simulink model "schSegwayArduino_2018a"  (R2018b)
settings: Solver=FixedStepDiscrete  StartTime=0.0  StopTime=inf  FixedStep=TECH  RelTol=1e-3  EnableMultiTasking=on
PreLoadFcn:
  | file:///C:/Users/maitrise/Documents/Elie/segwayEtudiant/segwayEtudiant/CzLeftRight.mat
InitFcn:
  | load CLeftRight.mat;
  | load  Kplace.mat
values from neighbouring files (symbols this model uses):
  K = [-22.0083946552 -0.385164851676 -3.66015572739 -0.971821179518]    [Kplace.mat]    (also in convertToParallelCells.m = 0; paralellCells.m = 0; programme_segway_etudiant.m = place(A,BUm,poles_BF))
  TECH = min(t(2:end)-t(1:(end-1)))    [drawScopeData.m]    (also in programme_segway_etudiant.m = 0.005)
  tfCLeftRight = tf(NumC,DenC)    [programme_segway_etudiant.m]
undefined symbols (not defined in the file or in its folder): denZ, numZ
libraries: arduinolib x7, cstblocks x1
settings Model: SimulationMode=external  ExtModeTrigDuration=2  Creator=KSURCT General  LastModifiedBy=maitrise
settings OptimizationCC: DefaultUnderspecifiedDataType=single  EnhancedBackFolding=on  PassReuseOutputArgsThreshold=0  MaxStackSize=64  OptimizeBlockOrder=speed  DifferentSizesBufferReuse=on  OptimizationCustomize=off
settings DebuggingCC: ParameterTunabilityLossMsg=error
settings HardwareCC: ProdBitPerPointer=32  ProdBitPerSizeT=32  ProdBitPerPtrDiffT=32  ProdLargestAtomicInteger=Long  ProdLargestAtomicFloat=Double  ProdWordSize=32  ProdHWDeviceType=ARM Compatible->ARM Cortex  UseEmbeddedCoderFeatures=off  UseSimulinkCoderFeatures=off
settings SFSimCC: MATLABDynamicMemAlloc=off
settings RTWCC: SystemTargetFile=ert.tlc  HardwareBoard=Arduino Due  TemplateMakefile=ert_default_tmf  GenerateReport=on  Toolchain=Arduino ARM  BuildConfiguration=Faster Runs  LaunchReport=on
settings CodeAppCC: ForceParamTrailComments=on  OperatorAnnotations=on  MangleLength=10
settings ERTTargetCC: ERTCustomFileBanners=off  SupportContinuousTime=on  SupportNonInlinedSFcns=on  RemoveResetFunc=off  SupportVariableSizeSignals=on  ModelStepFunctionPrototypeControlCompliant=off

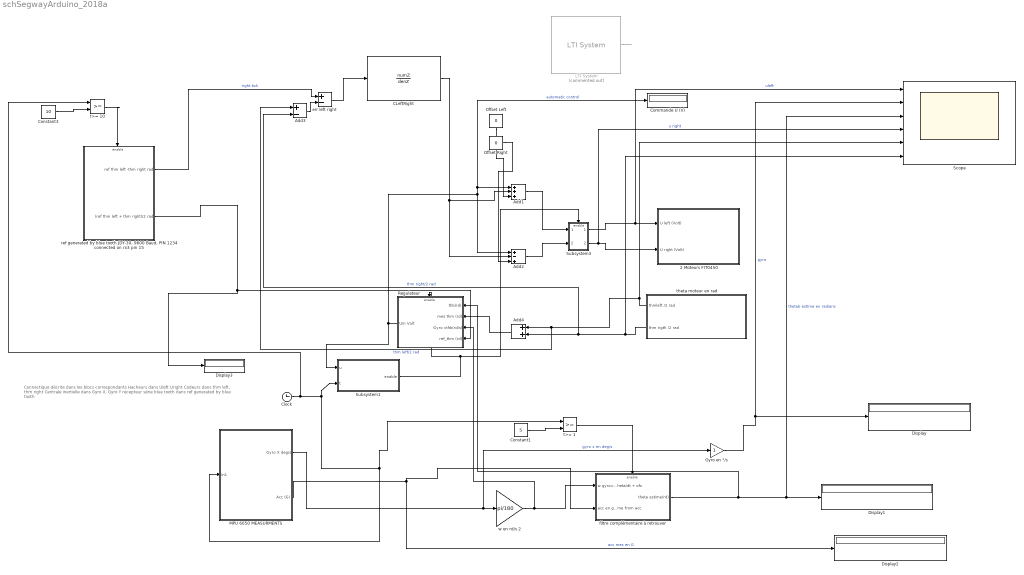
== system schSegwayArduino_2018a ==
  note: Connectique décrite dans les blocs correspondants
      | Hacheurs dans Uleft Uright
      | Codeurs dans thm left, thm right
      | Centrale inertielle dans Gyro X, Gyro Y
      | récepteur série blue tooth dans ref generated by blue tooth
  2 Moteurs FIT0450 : Subsystem
  Add1 : Sum  Inputs=+++
  Add2 : Sum  Inputs=+-+
  Add3 : Sum  Inputs=+-
  Add4 : Sum
  CLeftRight : DiscreteTransferFcn  Numerator=numZ  Denominator=denZ  SampleTime=TECH  mask(Tustin){tfP=tfCLeftRight, Tech=TECH}
      mask prompts: tfP "transfer Function F(p)"; Tech "Sample Time(s)"
      mask help:
      | discrete approximation (Tustin) of continuous transfer function
      | p -> 2/Te (z-1)/(z+1)
      mask init:
      | tfZ=c2d(tfP,Tech,'tustin');
      | [numZ,denZ]=tfdata(tfZ,'vector');
      mask Display: disp('F(p) \nTustin approx')
  Clock : Clock
  Commande U (V) : Display
  Constant1 : Constant  Value=5
  Constant3 : Constant  Value=10
  Display{,1..3} (4 alike) : Display
  Gyro en °/s : Gain
  LTI System : cstblocks/LTI System  Commented=on  sys=tf([1.42e2,2.36e3],[1,78])  IC=[]
  MPU 6050 MEASURMENTS : Subsystem
  "Offset Left " : Constant  Value=0
  Offset Right : Constant  Value=0
  Regulateur : Subsystem  TreatAsAtomicUnit=on
      settings: AttributesFormatString=REGULATEUR
  Scope : Scope  NumInputPorts=6
  Subsystem1 : Subsystem
  Subsystem3 : Subsystem
  err left right : Sum  Inputs=+-
  filtre complémentaire à retrouver : Subsystem
  "ref generated by blue tooth JDY-30, 9600 Baud, PIN 1234 connected on rx3 pin 15" : Subsystem
  t>= 1 : RelationalOperator  OutDataTypeStr=boolean  RndMeth=Simplest
  t>= 10 : RelationalOperator  OutDataTypeStr=boolean  RndMeth=Simplest
  theta moteur en rad : Subsystem
  w en rd/s 2 : Gain  Gain=pi/180
  wires:
  Subsystem1/1(enable) -> Subsystem3/Enable, Regulateur/Enable
  Add1/1 -> Subsystem3/1(In1)
  Add2/1 -> Subsystem3/2(In2)
  Subsystem3/1(Commande (V)) -> Scope/1, 2 Moteurs FIT0450/1(U left (Volt))  "uleft"
  Subsystem3/2(Commande (V)1) -> Scope/4, 2 Moteurs FIT0450/2(U right (Volt))  "u right"
  "ref generated by blue tooth JDY-30, 9600 Baud, PIN 1234 connected on rx3 pin 15"/2((ref thm left + thm right)/2 rad) -> Display3/1, Regulateur/4("ref_thm (rd) ")
  "ref generated by blue tooth JDY-30, 9600 Baud, PIN 1234 connected on rx3 pin 15"/1(ref thm left -thm right rad) -> err left right/1  "right tick"
  Regulateur/1(Um Volt) -> Commande U (V)/1, Add1/1, Add2/1, Subsystem1/1(u)  "automatic control"
  Clock/1 -> t>= 10/1, Subsystem1/2(t), t>= 1/1, MPU 6050 MEASURMENTS/1(In1)
  Gyro en °/s/1 -> Scope/2, Display/1  "gyro"
  CLeftRight/1 -> Add1/2, Add2/2
  t>= 10/1 -> "ref generated by blue tooth JDY-30, 9600 Baud, PIN 1234 connected on rx3 pin 15"/Enable
  Constant3/1 -> t>= 10/2
  theta moteur en rad/1(thmleft /2 rad) -> Scope/5, Add3/1, Add4/1  "thm left/2 rad"
  theta moteur en rad/2(thm rigth /2 rad) -> Scope/6, Add3/2, Add4/2  "thm right/2 rad"
  Add4/1 -> Regulateur/2(mes thm (rd))
  Add3/1 -> err left right/2
  "Offset Left "/1 -> Add1/3
  Offset Right/1 -> Add2/3
  filtre complémentaire à retrouver/1(theta estime(rd)) -> Regulateur/1(thb(rd)), Scope/3, Display1/1  "thetab estime en radians"
  MPU 6050 MEASURMENTS/1("Gyro X deg/s  ") -> Gyro en °/s/1, w en rd/s 2/1  "gyro x en deg/s"
  MPU 6050 MEASURMENTS/2(Acc (G)) -> Display2/1, filtre complémentaire à retrouver/2("acc en g = theta estime from acc ")  "acc mes en G"
  w en rd/s 2/1 -> Regulateur/3(Gyro vthb(rd/s)), filtre complémentaire à retrouver/1(w gyro=dtheta/dt + ofs)
  Constant1/1 -> t>= 1/2
  t>= 1/1 -> filtre complémentaire à retrouver/Enable
  LTI System/1 -> ?
  err left right/1 -> CLeftRight/1
  ? -> LTI System/1

== system schSegwayArduino_2018a/2 Moteurs FIT0450 ==
  note: CONNECTIQUE
      | Batterie de puissance : power Banc VoltCraft
      | brancher 2 resistances de 150 ohms 1/4 de watt en parallele sur la sortie 5V pour empecher la mise en pause
      | Hacheurs : MC33926 2,5 A et marche a 5V
      | Moteur droit FIT 0450U : Km=0,277 Nm/A , R=2,8ohm, Im=6e-3 kg m2 , fm =0.01 Nm/(rd/s)
      | Borne 39 Due sur In1 du pont en H
      | Borne 38 Due sur In2 du pont en H
      | Moteur gauche FIT 0450U
      | Borne 35 Due sur In1 du pont en H
      | Borne 34 Due sur In2 du pont en H
      | Moteurs droit et gauche
      | Fil noir moteurs sur out2 des ponts en H
      | Fil rouge moteurs sur out 1 des ponts en H
      | Gnd Due sur borne - (logique )
      | Gnd Alim Puissance sur borne - (puissance)
      | Vcc Alim Puissance 5V sur borne +, pas le 5v de la due, le 5v de puissance !
      | Codeur incremental moteur gauche (120.32 pas par tour)
      | fil rouge codeur sur 3,3V due ( surtout pas sur 5V : ATTENTION !... .)
      | fil noir codeur sur gnd due
      | fil bleu codeur sur borne 7 due
      | fil vert codeur sur borne 6 due
      | Codeur incremental moteur droit (120.32 pas par tour)
      | fil rouge codeur sur 3,3V due ( surtout pas sur 5V : ATTENTION !... .)
      | fil noir codeur sur gnd due
      | fil bleu codeur sur borne 4 due
      | fil vert codeur sur borne 3 due
  U left (Volt) : Inport
  U right (Volt) : Inport  Port=2
  Apply Command Pwm : Subsystem
  wires:
  U left (Volt)/1 -> Apply Command Pwm/1(U left (Volt))
  U right (Volt)/1 -> Apply Command Pwm/2(U right (Volt))

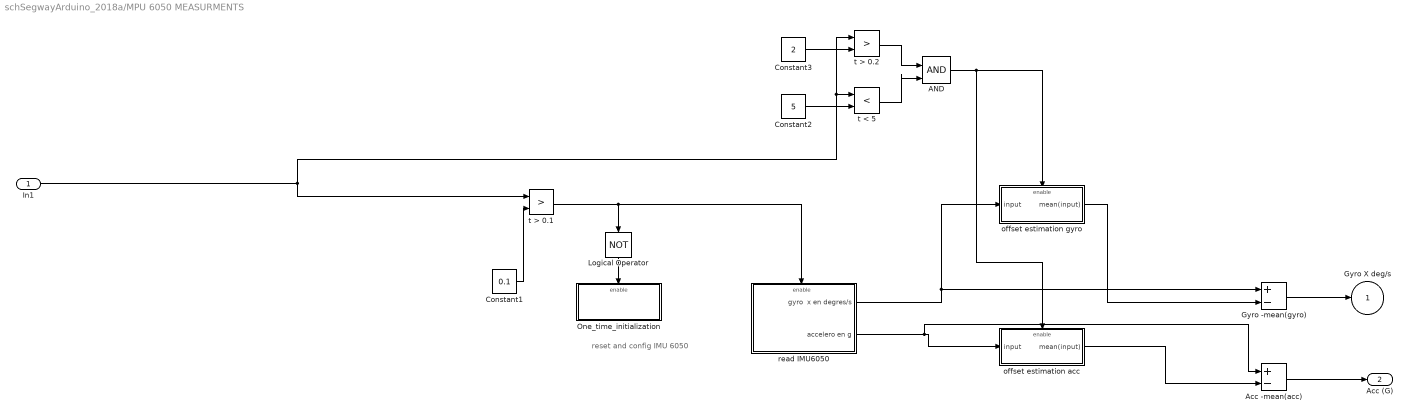
== system schSegwayArduino_2018a/MPU 6050 MEASURMENTS ==
  note: reset and config
      | IMU 6050
  In1 : Inport
  AND : Logic  IconShape=distinctive  AllPortsSameDT=off  OutDataTypeStr=boolean
  Acc -mean(acc) : Sum  Inputs=+-
  Constant1 : Constant  Value=0.1
  Constant2 : Constant  Value=5
  Constant3 : Constant  Value=2
  Gyro -mean(gyro) : Sum  Inputs=+-
  Logical Operator : Logic  Operator=NOT  AllPortsSameDT=off  OutDataTypeStr=boolean
  One_time_initialization : Subsystem  TreatAsAtomicUnit=on
  offset estimation acc : Subsystem  TreatAsAtomicUnit=on
  offset estimation gyro : Subsystem  TreatAsAtomicUnit=on
  read IMU6050 : Subsystem  TreatAsAtomicUnit=on
  t < 5 : RelationalOperator  Operator=<  OutDataTypeStr=boolean  RndMeth=Simplest
  t > 0.1 : RelationalOperator  Operator=>  OutDataTypeStr=boolean  RndMeth=Simplest
  t > 0.2 : RelationalOperator  Operator=>  OutDataTypeStr=boolean  RndMeth=Simplest
  "Gyro X deg/s  " : Outport
  Acc (G) : Outport  Port=2
  wires:
  t < 5/1 -> AND/2
  Logical Operator/1 -> One_time_initialization/Enable
  t > 0.1/1 -> read IMU6050/Enable, Logical Operator/1
  Gyro -mean(gyro)/1 -> "Gyro X deg/s  "/1
  Constant1/1 -> t > 0.1/2
  In1/1 -> t > 0.1/1, t > 0.2/1, t < 5/1
  AND/1 -> offset estimation acc/Enable, offset estimation gyro/Enable
  offset estimation gyro/1(mean(input)) -> Gyro -mean(gyro)/2
  read IMU6050/1(gyro  x en degres/s) -> offset estimation gyro/1(input), Gyro -mean(gyro)/1
  t > 0.2/1 -> AND/1
  Constant2/1 -> t < 5/2
  Constant3/1 -> t > 0.2/2
  read IMU6050/2(accelero en g) -> Acc -mean(acc)/1, offset estimation acc/1(input)
  offset estimation acc/1(mean(input)) -> Acc -mean(acc)/2
  Acc -mean(acc)/1 -> Acc (G)/1

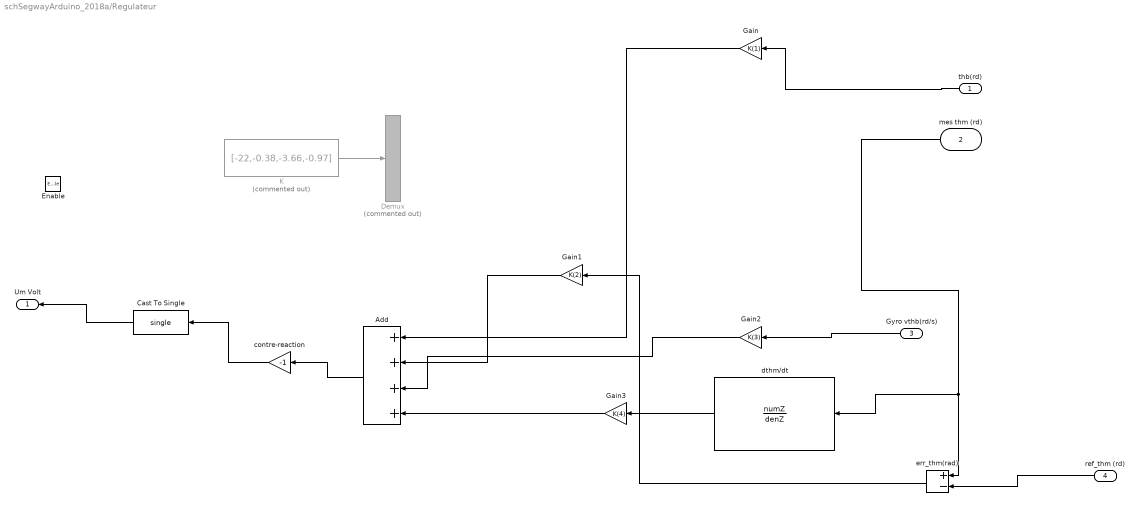
== system schSegwayArduino_2018a/Regulateur ==
  thb(rd) : Inport
  mes thm (rd) : Inport  Port=2
  Gyro vthb(rd/s) : Inport  Port=3
  "ref_thm (rd) " : Inport  Port=4
  Enable : EnablePort  StatesWhenEnabling=reset
  Add : Sum  Inputs=++++
  Cast To Single : DataTypeConversion  OutDataTypeStr=single
  Demux : Demux  Commented=on
  Gain : Gain  Gain=K(1)
  Gain1 : Gain  Gain=K(2)
  Gain2 : Gain  Gain=K(3)
  Gain3 : Gain  Gain=K(4)
  K : Constant  Commented=on  Value=[-22,-0.38,-3.66,-0.97]
  contre-reaction : Gain  Gain=-1
  dthm/dt : DiscreteTransferFcn  Numerator=numZ  Denominator=denZ  SampleTime=TECH  mask(Tustin){tfP=tf([1,0],[0.01,1]), Tech=TECH}
      mask prompts: tfP "transfer Function F(p)"; Tech "Sample Time(s)"
      mask help:
      | discrete approximation (Tustin) of continuous transfer function
      | p -> 2/Te (z-1)/(z+1)
      mask init:
      | tfZ=c2d(tfP,Tech,'tustin');
      | [numZ,denZ]=tfdata(tfZ,'vector');
      mask Display: disp('F(p) \nTustin approx')
  err_thm(rad) : Sum  Inputs=+-
  Um Volt : Outport  OutputWhenDisabled=reset  InitialOutput=0
  wires:
  Cast To Single/1 -> Um Volt/1
  mes thm (rd)/1 -> dthm/dt/1, err_thm(rad)/1
  thb(rd)/1 -> Gain/1
  dthm/dt/1 -> Gain3/1
  Gain3/1 -> Add/4
  Gain2/1 -> Add/3
  Add/1 -> contre-reaction/1
  contre-reaction/1 -> Cast To Single/1
  K/1 -> Demux/1
  Gain1/1 -> Add/2
  Gain/1 -> Add/1
  "ref_thm (rd) "/1 -> err_thm(rad)/2
  err_thm(rad)/1 -> Gain1/1
  Gyro vthb(rd/s)/1 -> Gain2/1

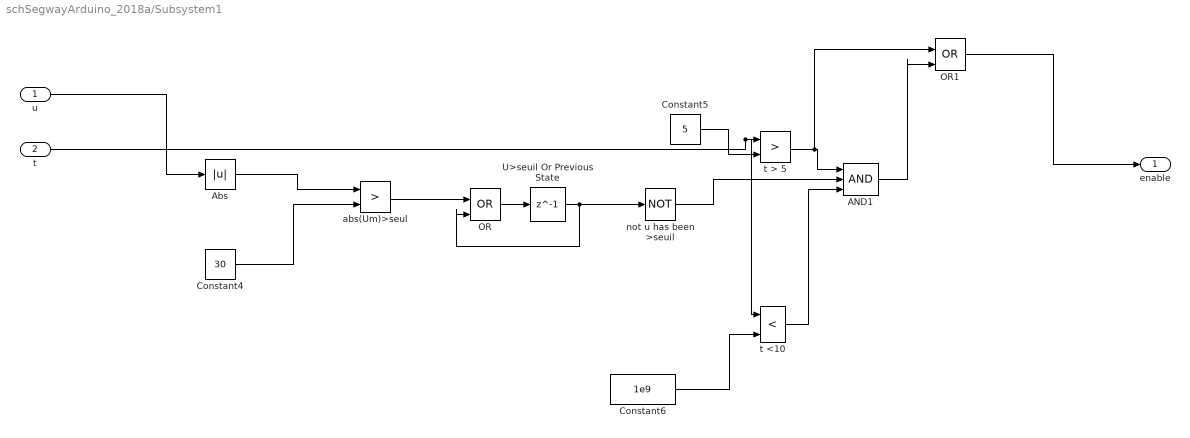
== system schSegwayArduino_2018a/Subsystem1 ==
  u : Inport
  t : Inport  Port=2
  AND1 : Logic  Inputs=3  IconShape=distinctive  AllPortsSameDT=off  OutDataTypeStr=boolean
  Abs : Abs
  Constant4 : Constant  Value=30
  Constant5 : Constant  Value=5
  Constant6 : Constant  Value=1e9
  OR : Logic  Operator=OR  IconShape=distinctive  AllPortsSameDT=off  OutDataTypeStr=boolean
  OR1 : Logic  Operator=OR  IconShape=distinctive  AllPortsSameDT=off  OutDataTypeStr=boolean
  U>seuil Or Previous State : Delay  DelayLength=1  InitialCondition=0  SampleTime=TECH
  abs(Um)>seul : RelationalOperator  Operator=>  OutDataTypeStr=boolean  RndMeth=Simplest
  not u has been >seuil : Logic  Operator=NOT  IconShape=distinctive  AllPortsSameDT=off  OutDataTypeStr=boolean
  t <10 : RelationalOperator  Operator=<  OutDataTypeStr=boolean  RndMeth=Simplest
  t > 5 : RelationalOperator  Operator=>  OutDataTypeStr=boolean  RndMeth=Simplest
  enable : Outport
  wires:
  Constant4/1 -> abs(Um)>seul/2
  not u has been >seuil/1 -> AND1/2
  Constant6/1 -> t <10/2
  abs(Um)>seul/1 -> OR/1
  t/1 -> t <10/1, t > 5/1
  u/1 -> Abs/1
  OR/1 -> U>seuil Or Previous State/1
  t > 5/1 -> OR1/1, AND1/1
  t <10/1 -> AND1/3
  Constant5/1 -> t > 5/2
  U>seuil Or Previous State/1 -> OR/2, not u has been >seuil/1
  Abs/1 -> abs(Um)>seul/1
  OR1/1 -> enable/1
  AND1/1 -> OR1/2

== system schSegwayArduino_2018a/Subsystem3 ==
  In1 : Inport
  In2 : Inport  Port=2
  Enable : EnablePort
  U_left limited(V) : Saturate  UpperLimit=5  LowerLimit=-5
  U_right limited(V) : Saturate  UpperLimit=5  LowerLimit=-5
  Commande (V) : Outport  OutputWhenDisabled=reset  InitialOutput=0
  Commande (V)1 : Outport  Port=2  OutputWhenDisabled=reset  InitialOutput=0
  wires:
  U_right limited(V)/1 -> Commande (V)1/1  "Commande (V)"
  In1/1 -> U_left limited(V)/1
  In2/1 -> U_right limited(V)/1
  U_left limited(V)/1 -> Commande (V)/1  "Commande (V)"

== system schSegwayArduino_2018a/filtre complémentaire à retrouver ==
  note: travail a realiser : creer votre propre schema de filtre complementaire de cte de temps tauFlt=1s
      | principe: on peut estimer theta de 2 facons
      | 1- en integrant la vitesse mesure wgyro =dtheta/dt +offset, ce qui fournit une bonne estimation pour les variations rapides , mais dérive au cours du temps , car on integre aussi l'offset du gyro
      | 2- en employant l'acceleration mesuree suivant l'axe x de l'accelerometre: acc= g.sin(theta) + acceleration segway suivant x, soit approximativement acc = g.theta + acceleration propre suivant x
      | Comme en moyenne le segway n'accélère pas, la moyenne de cette mesure (en g) obtenue par filtrage passe-bas fournit une bonne approximation des variations lentes de theta
      |
      | Equations et filtre complementaire :
      | Notations Acc = acc mesuree en G , w Gyro = dtheta/dt mesuree avec le gyro , thetaest= theta estime, et on raisonne dans le domaine symbolique de Laplace :
      | On peut idealment estimer theta avec la formule suivante :
      | Theta estime(p) = ( 1+ tau.p )/(1+tau.p) Theta(p) =[ 1/ (1+Tau.p) . theta(p) ] + [ tau .p / (1+tau. p) ] .( 1/p ) [p.theta(p) ]
      | en fabriquant le premier terme de l'addition depuis la mesure de l'accéléromètre exprimee en g, et la seconde partie depuis la mesure du gyroscope, on obtient bien l'effet escompté :
      | Theta estime(p) = [ passebas ] . acc en g + [passe-haut ] . intégrale du gyro
      |
      | 1- l'accéléromètre est passé au travers d'un passe-bas qui en extrait la valeur moyenne en éliminant les variations rapides
      | 2- l'intégrale du gyro est passée au travers d'un passe-haut qui élimine la dérrive due à l'offset
      |
      | Techniquement il est stupide d'integrer le gyroscope pour le dériver juste ensuite, on programme donc :
      | Theta estime (p) = [ 1/ (1+Tau.p) ] [ Acc(p) en g + tau . [wgyro(p) = p.theta(p) +offset ]
      | soit encore
      | Theta estime = passe bas de constante de temps tau . [acc en g + tau . gyro]
      | C'est ce schema que l'on vous demande de réaliser, avec tau = 1s , que vous pourrez eventuellement adapter par la suite
  w gyro=dtheta/dt + ofs : Inport
  "acc en g = theta estime from acc " : Inport  Port=2
  Enable : EnablePort
  Filtre complementaire (Tustin approx) : Subsystem  mask{tauFlt=2}
      mask prompts: tauFlt "cte de tps (s)"
      mask Display: disp('filtre complementaire\nde cte de temps ajustable');
  low pass filter : DiscreteTransferFcn  Commented=on  Numerator=numZ  Denominator=denZ  SampleTime=TECH  mask(Tustin){tfP=tf(1,1), Tech=TECH}
      mask prompts: tfP "transfer Function F(p)"; Tech "Sample Time(s)"
      mask help:
      | discrete approximation (Tustin) of continuous transfer function
      | p -> 2/Te (z-1)/(z+1)
      mask init:
      | tfZ=c2d(tfP,Tech,'tustin');
      | [numZ,denZ]=tfdata(tfZ,'vector');
      mask Display: disp('F(p) \nTustin approx')
  theta estime(rd) : Outport  VectorParamsAs1DForOutWhenUnconnected=on
  wires:
  "acc en g = theta estime from acc "/1 -> Filtre complementaire (Tustin approx)/2("acc /g = theta estime ")
  Filtre complementaire (Tustin approx)/1(theta estime(rd)) -> theta estime(rd)/1
  w gyro=dtheta/dt + ofs/1 -> Filtre complementaire (Tustin approx)/1(w gyro=dtheta/dt + ofs)

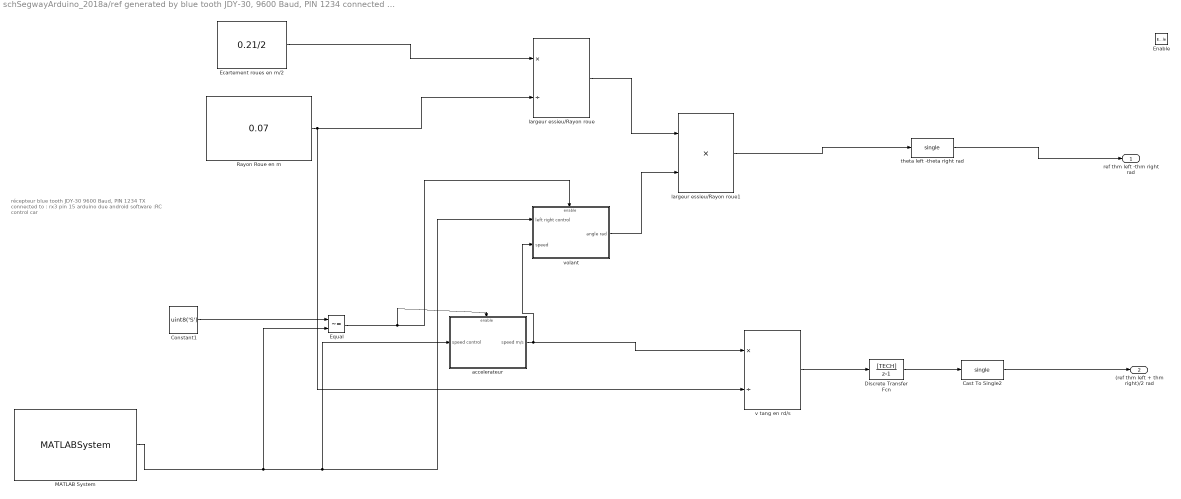
== system schSegwayArduino_2018a/ref generated by blue tooth JDY-30, 9600 Baud, PIN 1234 connected on rx3 pin 15 ==
  note: récepteur blue tooth JDY-30
      | 9600 Baud,
      | PIN 1234
      | TX connected to : rx3 pin 15 arduino due
      | android software :RC control car
  Enable : EnablePort
  Cast To Single2 : DataTypeConversion  OutDataTypeStr=single
  Constant1 : Constant  Value=uint8('S')
  Discrete Transfer Fcn : DiscreteTransferFcn  Numerator=[TECH]  Denominator=[1 -1]  SampleTime=TECH  OutDataTypeStr=Inherit: Same as input
  Ecartement roues en m/2 : Constant  Value=0.21/2
  Equal : RelationalOperator  Operator=~=  OutDataTypeStr=boolean  RndMeth=Simplest
  MATLAB System : MATLABSystem  System=SerialRead  id=3  baudRate=9600  SampleTime=TECH
      mask Type: SerialRead
      mask Display:
      | disp(['serial Read :' char(10) 'Serial,Serial1,Serial2,Serial3' char(10) 'depending on id: [0..3]' char(10) '']);
      | port_label('output',1,'value');
  Rayon Roue en m : Constant  Value=0.07
  accelerateur : Subsystem
  largeur essieu/Rayon roue : Product  Inputs=*/
  largeur essieu/Rayon roue1 : Product  Inputs=**
  theta left -theta right rad : DataTypeConversion  OutDataTypeStr=single
  v tang en rd/s : Product  Inputs=*/
  volant : Subsystem
  ref thm left -thm right rad : Outport
  (ref thm left + thm right)/2 rad : Outport  Port=2
  wires:
  Discrete Transfer Fcn/1 -> Cast To Single2/1
  v tang en rd/s/1 -> Discrete Transfer Fcn/1
  Ecartement roues en m/2/1 -> largeur essieu/Rayon roue/1
  largeur essieu/Rayon roue/1 -> largeur essieu/Rayon roue1/1
  largeur essieu/Rayon roue1/1 -> theta left -theta right rad/1
  theta left -theta right rad/1 -> ref thm left -thm right rad/1
  Cast To Single2/1 -> (ref thm left + thm right)/2 rad/1
  Rayon Roue en m/1 -> largeur essieu/Rayon roue/2, v tang en rd/s/2
  accelerateur/1(speed m/s) -> volant/2(speed), v tang en rd/s/1
  volant/1(angle rad) -> largeur essieu/Rayon roue1/2
  Constant1/1 -> Equal/1
  Equal/1 -> volant/Enable, accelerateur/Enable
  MATLAB System/1 -> accelerateur/1(speed control), volant/1(left right control), Equal/2

== system schSegwayArduino_2018a/theta moteur en rad ==
  note: CONNECTIQUE
      | Hacheurs : MC
      | Moteur droit FIT 0450U
      | Borne 39 Due sur In1 du pont en H
      | Borne 38 Due sur In2 du pont en H
      | Moteur gauche FIT 0450U
      | Borne 35 Due sur In1 du pont en H
      | Borne 34 Due sur In2 du pont en H
      | Moteurs droit et gauche
      | Fil noir moteurs sur out2 des ponts en H
      | Fil rouge moteurs sur out 1 des ponts en H
      | Gnd Due sur borne - (logique )
      | Gnd Alim Puissance sur borne - (puissance)
      | Vcc Alim Puissance 5V sur borne +, pas le 5v de la due, le 5v de puissance !
      | Codeur incremental moteur gauche (120.32 pas par tour)
      | fil rouge codeur sur 3,3V due ( surtout pas sur 5V : ATTENTION !... .)
      | fil noir codeur sur gnd due
      | fil bleu codeur sur borne 7 due
      | fil vert codeur sur borne 6 due
      | Codeur incremental moteur droit (120.32 pas par tour)
      | fil rouge codeur sur 3,3V due ( surtout pas sur 5V : ATTENTION !... .)
      | fil noir codeur sur gnd due
      | fil bleu codeur sur borne 4 due
      | fil vert codeur sur borne 3 due
  Cast To Single : DataTypeConversion  OutDataTypeStr=single
  Cast To Single1 : DataTypeConversion  OutDataTypeStr=single
  left Encoder : MATLABSystem  System=EncoderRead  pinA=uint8( 7 )  pinB=uint8( 6 )  id=uint8( 1 )  SampleTime=TECH
      mask Type: EncoderRead
      mask Display:
      | disp('encoder');
      | port_label('output',1,'ticks');
  rightEncoder : MATLABSystem  System=EncoderRead  pinA=uint8( 3 )  pinB=uint8( 4 )  id=uint8( 0 )  SampleTime=TECH
      mask Type: EncoderRead
      mask Display:
      | disp('encoder');
      | port_label('output',1,'ticks');
  thm left/2 : Gain  Gain=1/2 * (2*pi/(120*32))
  thm right /2 : Gain  Gain=1/2 * (2*pi/(120*32))
  thmleft /2 rad : Outport
  thm rigth /2 rad : Outport  Port=2
  wires:
  Cast To Single/1 -> thm left/2/1
  Cast To Single1/1 -> thm right /2/1
  thm right /2/1 -> thm rigth /2 rad/1
  thm left/2/1 -> thmleft /2 rad/1
  rightEncoder/1 -> Cast To Single1/1
  left Encoder/1 -> Cast To Single/1

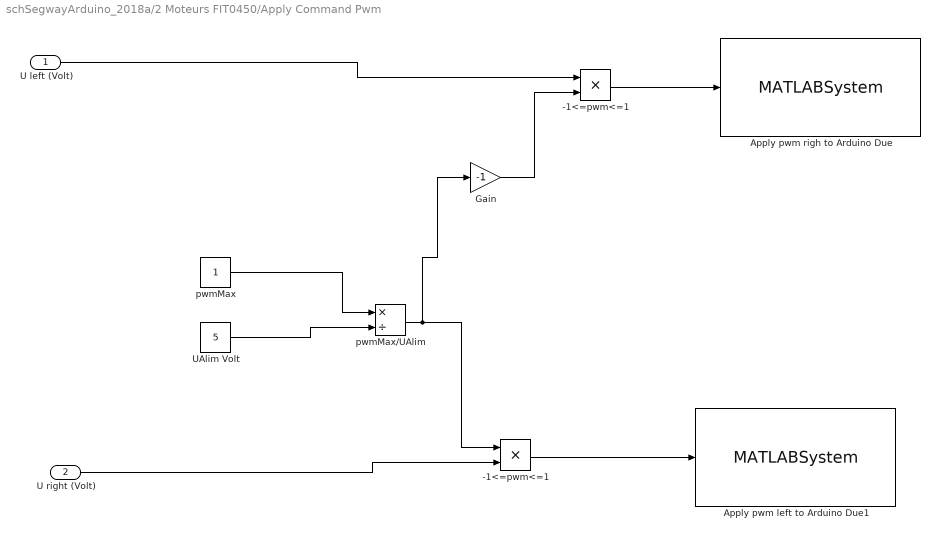
== system schSegwayArduino_2018a/2 Moteurs FIT0450/Apply Command Pwm ==
  U left (Volt) : Inport
  U right (Volt) : Inport  Port=2
  -1<=pwm<=1 : Product  Inputs=**
  "-1<=pwm<=1 " : Product  Inputs=**
  Apply pwm left to Arduino Due1 : MATLABSystem  System=PwmWrite  pin=38  useComplementaryPin=1  periodMicros=50  id=1  SampleTime=TECH
      mask Type: PwmWrite
      mask Display:
      | disp(['-1<=Pwm<=1' char(10) 'pins : 6,9' char(10) '7-45,8-44,34-35,36-37,38-39,40-41']);
      | port_label('input',1,'u');
  Apply pwm righ to Arduino Due : MATLABSystem  System=PwmWrite  pin=34  useComplementaryPin=1  periodMicros=50  id=0  SampleTime=TECH
      mask Type: PwmWrite
      mask Display:
      | disp(['-1<=Pwm<=1' char(10) 'pins : 6,9' char(10) '7-45,8-44,34-35,36-37,38-39,40-41']);
      | port_label('input',1,'u');
  Gain : Gain  Gain=-1
  UAlim Volt : Constant  Value=5
  pwmMax : Constant
  pwmMax/UAlim : Product  Inputs=*/
  wires:
  UAlim Volt/1 -> pwmMax/UAlim/2
  pwmMax/1 -> pwmMax/UAlim/1
  U right (Volt)/1 -> -1<=pwm<=1/2
  U left (Volt)/1 -> "-1<=pwm<=1 "/1
  pwmMax/UAlim/1 -> -1<=pwm<=1/1, Gain/1
  -1<=pwm<=1/1 -> Apply pwm left to Arduino Due1/1
  "-1<=pwm<=1 "/1 -> Apply pwm righ to Arduino Due/1
  Gain/1 -> "-1<=pwm<=1 "/2

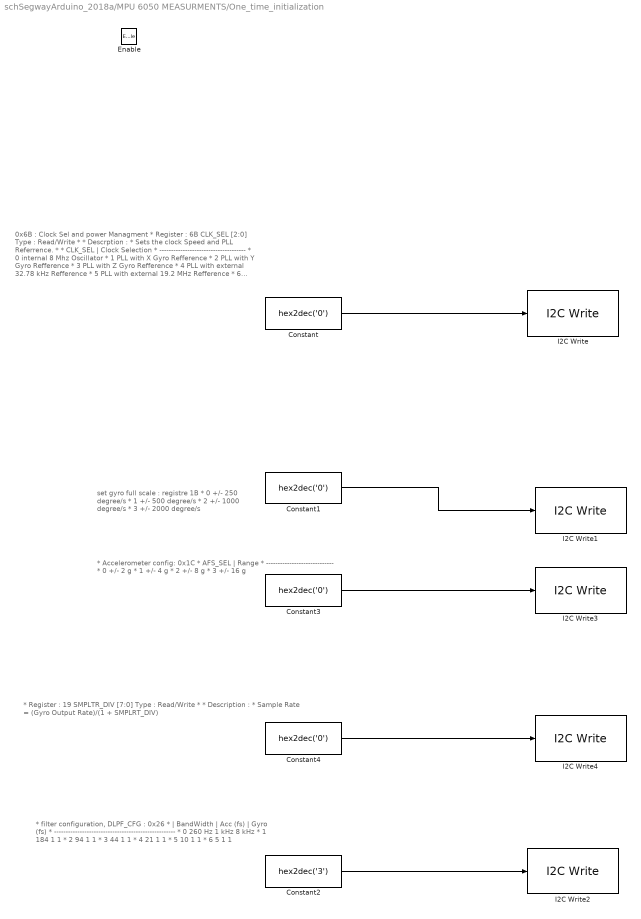
== system schSegwayArduino_2018a/MPU 6050 MEASURMENTS/One_time_initialization ==
  note: *  Register : 19          SMPLTR_DIV [7:0]       Type :  Read/Write
      |      *
      |      *  Description :
      |      *    Sample Rate = (Gyro Output Rate)/(1 + SMPLRT_DIV)
  note: * filter configuration, DLPF_CFG : 0x26
      |      *         |    BandWidth  |   Acc (fs)  |  Gyro (fs)
      |      *    ----------------------------------------------------
      |      *        0             260 Hz          1 kHz       8 kHz
      |      *        1             184             1           1
      |      *        2              94             1           1
      |      *        3              44             1           1
      |      *        4              21             1           1
      |      *        5              10             1           1
      |      *        6               5             1           1
  note: set gyro full scale : registre 1B
      |      *              0         +/- 250 degree/s
      |      *              1         +/- 500 degree/s
      |      *              2         +/- 1000 degree/s
      |      *              3         +/- 2000 degree/s
  note: * Accelerometer config: 0x1C
      |   *           AFS_SEL    |     Range
      |      *          -----------------------------
      |      *              0            +/- 2 g
      |      *              1            +/- 4 g
      |      *              2            +/- 8 g
      |      *              3            +/- 16 g
  note: 0x6B : Clock Sel and power Managment
      | * Register : 6B CLK_SEL [2:0] Type : Read/Write
      | *
      | * Descrption :
      | * Sets the clock Speed and PLL Referrence.
      | *
      | * CLK_SEL | Clock Selection
      | * -------------------------------------
      | * 0 internal 8 Mhz Oscillator
      | * 1 PLL with X Gyro Refference
      | * 2 PLL with Y Gyro Refference
      | * 3 PLL with Z Gyro Refference
      | * 4 PLL with external 32.78 kHz Refference
      | * 5 PLL with external 19.2 MHz Refference
      | * 6 Reserved
      | * 7 Stops and puts to sleep.
      | *
      | * SLEEP [bit 6] - set '1' to put MPU 6050 to Sleep.
      | * CYCLE [bit 5] - set '1' and Sleep is disabled.
      | * TEMP_DIS [bit 3] - set '1' to disable Temp. Sensor
      | * DEV_RESET [bit 7] - set to '1' to reset the internal Register.
  Enable : EnablePort
  Constant{,1,3..4} (4 alike) : Constant  Value=hex2dec('0')  OutDataTypeStr=uint8
  Constant2 : Constant  Value=hex2dec('3')  OutDataTypeStr=uint8
  I2C Write : arduinolib/I2C Write  Priority=1  I2CModule=0  Mode=Master  SlaveAddress=hex2dec( '68' )  SlaveByteOrder=BigEndian  Direction=Transmitter  RegisterAddressMode=on  RegisterAddress=hex2dec( '6B' )  SlaveDataType=uint16  DataLength=1  NoAck=off  RepeatedStart=off  OutputStatus=off  blockPlatform=arduino
      settings: AttributesFormatString=Priority=%<Priority>  SourceProductBaseCode=ARDUINO
  I2C Write1 : arduinolib/I2C Write  Priority=2  I2CModule=0  Mode=Master  SlaveAddress=hex2dec( '68' )  SlaveByteOrder=BigEndian  Direction=Transmitter  RegisterAddressMode=on  RegisterAddress=hex2dec( '1B' )  SlaveDataType=uint16  DataLength=1  NoAck=off  RepeatedStart=off  OutputStatus=off  blockPlatform=arduino
      settings: AttributesFormatString=Priority=%<Priority>  SourceProductBaseCode=ARDUINO
  I2C Write2 : arduinolib/I2C Write  Priority=5  I2CModule=0  Mode=Master  SlaveAddress=hex2dec( '68' )  SlaveByteOrder=BigEndian  Direction=Transmitter  RegisterAddressMode=on  RegisterAddress=hex2dec( '26' )  SlaveDataType=uint16  DataLength=1  NoAck=off  RepeatedStart=off  OutputStatus=off  blockPlatform=arduino
      settings: AttributesFormatString=Priority=%<Priority>  SourceProductBaseCode=ARDUINO
  I2C Write3 : arduinolib/I2C Write  Priority=3  I2CModule=0  Mode=Master  SlaveAddress=hex2dec( '68' )  SlaveByteOrder=BigEndian  Direction=Transmitter  RegisterAddressMode=on  RegisterAddress=hex2dec( '1C' )  SlaveDataType=uint16  DataLength=1  NoAck=off  RepeatedStart=off  OutputStatus=off  blockPlatform=arduino
      settings: AttributesFormatString=Priority=%<Priority>  SourceProductBaseCode=ARDUINO
  I2C Write4 : arduinolib/I2C Write  Priority=4  I2CModule=0  Mode=Master  SlaveAddress=hex2dec( '68' )  SlaveByteOrder=BigEndian  Direction=Transmitter  RegisterAddressMode=on  RegisterAddress=hex2dec( '19' )  SlaveDataType=uint16  DataLength=1  NoAck=off  RepeatedStart=off  OutputStatus=off  blockPlatform=arduino
      settings: AttributesFormatString=Priority=%<Priority>  SourceProductBaseCode=ARDUINO
  wires:
  Constant/1 -> I2C Write/1
  Constant1/1 -> I2C Write1/1
  Constant2/1 -> I2C Write2/1
  Constant3/1 -> I2C Write3/1
  Constant4/1 -> I2C Write4/1

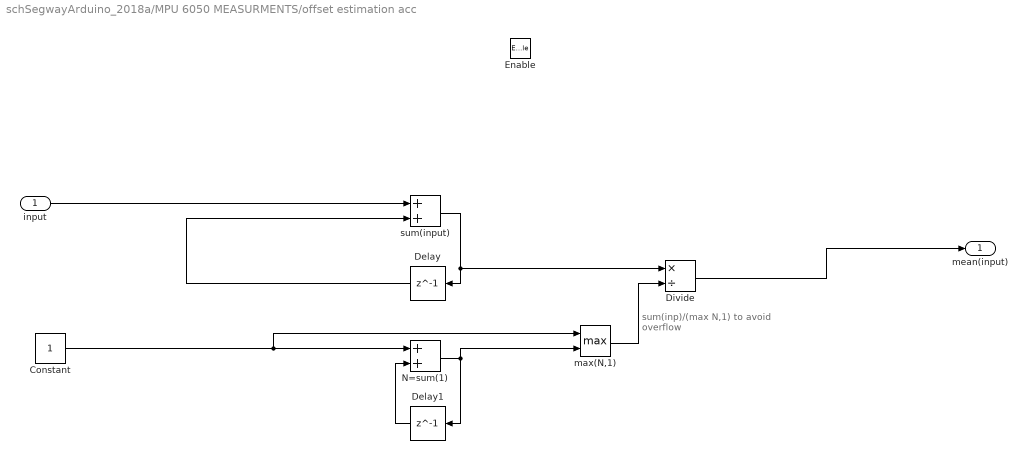
== system schSegwayArduino_2018a/MPU 6050 MEASURMENTS/offset estimation acc ==
  note: sum(inp)/(max N,1)
      | to avoid overflow
  input : Inport
  Enable : EnablePort
  Constant : Constant
  Delay : Delay  DelayLength=1  SampleTime=TECH
  Delay1 : Delay  DelayLength=1  SampleTime=TECH
  Divide : Product  Inputs=*/
  N=sum(1) : Sum
  max(N,1) : MinMax  Function=max  Inputs=2
  sum(input) : Sum
  mean(input) : Outport  InitialOutput=0
  wires:
  sum(input)/1 -> Delay/1, Divide/1
  Delay/1 -> sum(input)/2
  input/1 -> sum(input)/1
  N=sum(1)/1 -> Delay1/1, max(N,1)/2
  Delay1/1 -> N=sum(1)/2
  Constant/1 -> max(N,1)/1, N=sum(1)/1
  max(N,1)/1 -> Divide/2
  Divide/1 -> mean(input)/1

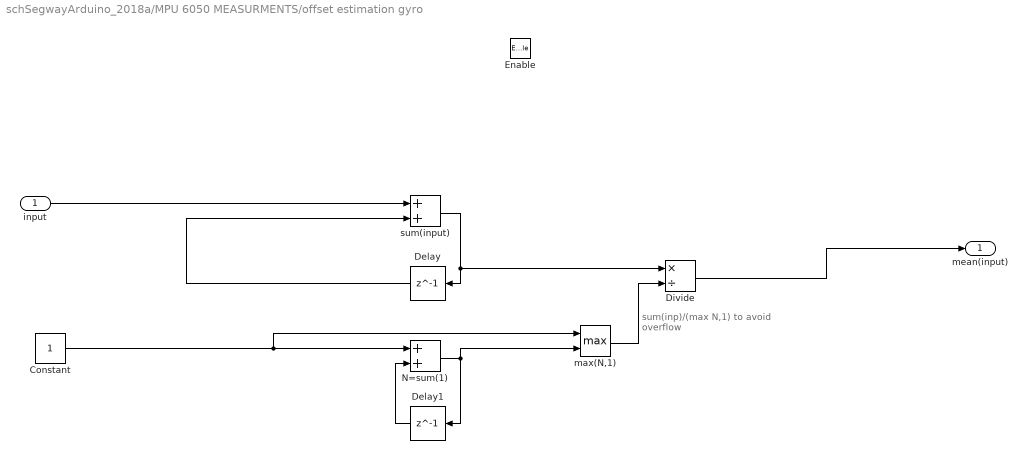
== system schSegwayArduino_2018a/MPU 6050 MEASURMENTS/offset estimation gyro ==
  note: sum(inp)/(max N,1)
      | to avoid overflow
  input : Inport
  Enable : EnablePort
  Constant : Constant
  Delay : Delay  DelayLength=1  SampleTime=TECH
  Delay1 : Delay  DelayLength=1  SampleTime=TECH
  Divide : Product  Inputs=*/
  N=sum(1) : Sum
  max(N,1) : MinMax  Function=max  Inputs=2
  sum(input) : Sum
  mean(input) : Outport  InitialOutput=0
  wires:
  sum(input)/1 -> Delay/1, Divide/1
  Delay/1 -> sum(input)/2
  input/1 -> sum(input)/1
  N=sum(1)/1 -> Delay1/1, max(N,1)/2
  Delay1/1 -> N=sum(1)/2
  Constant/1 -> max(N,1)/1, N=sum(1)/1
  max(N,1)/1 -> Divide/2
  Divide/1 -> mean(input)/1

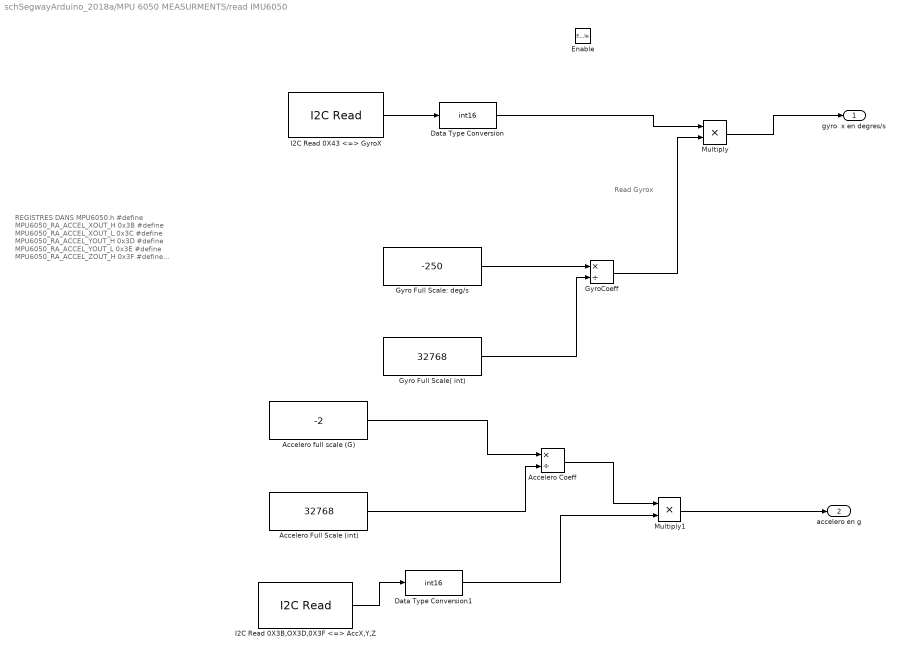
== system schSegwayArduino_2018a/MPU 6050 MEASURMENTS/read IMU6050 ==
  note: REGISTRES DANS MPU6050.h
      | #define MPU6050_RA_ACCEL_XOUT_H     0x3B
      | #define MPU6050_RA_ACCEL_XOUT_L     0x3C
      | #define MPU6050_RA_ACCEL_YOUT_H     0x3D
      | #define MPU6050_RA_ACCEL_YOUT_L     0x3E
      | #define MPU6050_RA_ACCEL_ZOUT_H     0x3F
      | #define MPU6050_RA_ACCEL_ZOUT_L     0x40
      | #define MPU6050_RA_TEMP_OUT_H       0x41
      | #define MPU6050_RA_TEMP_OUT_L       0x42
      | #define MPU6050_RA_GYRO_XOUT_H      0x43
      | #define MPU6050_RA_GYRO_XOUT_L      0x44
      | #define MPU6050_RA_GYRO_YOUT_H      0x45
      | #define MPU6050_RA_GYRO_YOUT_L      0x46
      | #define MPU6050_RA_GYRO_ZOUT_H      0x47
      | #define MPU6050_RA_GYRO_ZOUT_L      0x48
  note: Read Gyrox
  Enable : EnablePort
  Accelero Coeff : Product  Inputs=*/  OutDataTypeStr=single
  Accelero Full Scale (int) : Constant  Value=32768
  Accelero full scale (G) : Constant  Value=-2
  Data Type Conversion : DataTypeConversion  OutDataTypeStr=int16  ConvertRealWorld=Stored Integer (SI)
  Data Type Conversion1 : DataTypeConversion  OutDataTypeStr=int16  ConvertRealWorld=Stored Integer (SI)
  Gyro Full Scale( int) : Constant  Value=32768
  Gyro Full Scale: deg/s : Constant  Value=-250
  GyroCoeff : Product  Inputs=*/  OutDataTypeStr=single
  I2C Read 0X3B,OX3D,0X3F <=> AccX,Y,Z : arduinolib/I2C Read  Priority=2  I2CModule=0  Mode=Master  SlaveAddress=hex2dec( '68' )  SlaveByteOrder=BigEndian  Direction=Receiver  RegisterAddressMode=on  RegisterAddress=hex2dec( '3F' )  SlaveDataType=uint16  DataLength=1  NoAck=off  RepeatedStart=off  OutputStatus=off  blockPlatform=arduino  SampleTime=TECH
      settings: SourceProductBaseCode=ARDUINO
  I2C Read 0X43 <=> GyroX : arduinolib/I2C Read  Priority=1  I2CModule=0  Mode=Master  SlaveAddress=hex2dec( '68' )  SlaveByteOrder=BigEndian  Direction=Receiver  RegisterAddressMode=on  RegisterAddress=hex2dec( '43' )  SlaveDataType=uint16  DataLength=1  NoAck=off  RepeatedStart=off  OutputStatus=off  blockPlatform=arduino  SampleTime=TECH
      settings: SourceProductBaseCode=ARDUINO
  Multiply : Product
  Multiply1 : Product
  gyro  x en degres/s : Outport  InitialOutput=0
  accelero en g : Outport  Port=2  InitialOutput=0
  wires:
  I2C Read 0X43 <=> GyroX/1 -> Data Type Conversion/1
  Data Type Conversion/1 -> Multiply/1
  Multiply/1 -> gyro  x en degres/s/1
  Gyro Full Scale: deg/s/1 -> GyroCoeff/1
  Gyro Full Scale( int)/1 -> GyroCoeff/2
  GyroCoeff/1 -> Multiply/2
  I2C Read 0X3B,OX3D,0X3F <=> AccX,Y,Z/1 -> Data Type Conversion1/1
  Data Type Conversion1/1 -> Multiply1/2
  Multiply1/1 -> accelero en g/1
  Accelero Coeff/1 -> Multiply1/1
  Accelero Full Scale (int)/1 -> Accelero Coeff/2
  Accelero full scale (G)/1 -> Accelero Coeff/1

== system schSegwayArduino_2018a/filtre complémentaire à retrouver/Filtre complementaire (Tustin approx) ==
  w gyro=dtheta/dt + ofs : Inport
  "acc /g = theta estime " : Inport  Port=2
  Add : Sum
  Gain : Gain  Gain=tauFlt
  low pass filter : DiscreteTransferFcn  Numerator=numZ  Denominator=denZ  SampleTime=TECH  mask(Tustin){tfP=tf(1,[tauFlt,1]), Tech=TECH}
      mask prompts: tfP "transfer Function F(p)"; Tech "Sample Time(s)"
      mask help:
      | discrete approximation (Tustin) of continuous transfer function
      | p -> 2/Te (z-1)/(z+1)
      mask init:
      | tfZ=c2d(tfP,Tech,'tustin');
      | [numZ,denZ]=tfdata(tfZ,'vector');
      mask Display: disp('F(p) \nTustin approx')
  theta estime(rd) : Outport  VectorParamsAs1DForOutWhenUnconnected=on
  wires:
  w gyro=dtheta/dt + ofs/1 -> Gain/1
  Gain/1 -> Add/1
  "acc /g = theta estime "/1 -> Add/2
  Add/1 -> low pass filter/1
  low pass filter/1 -> theta estime(rd)/1

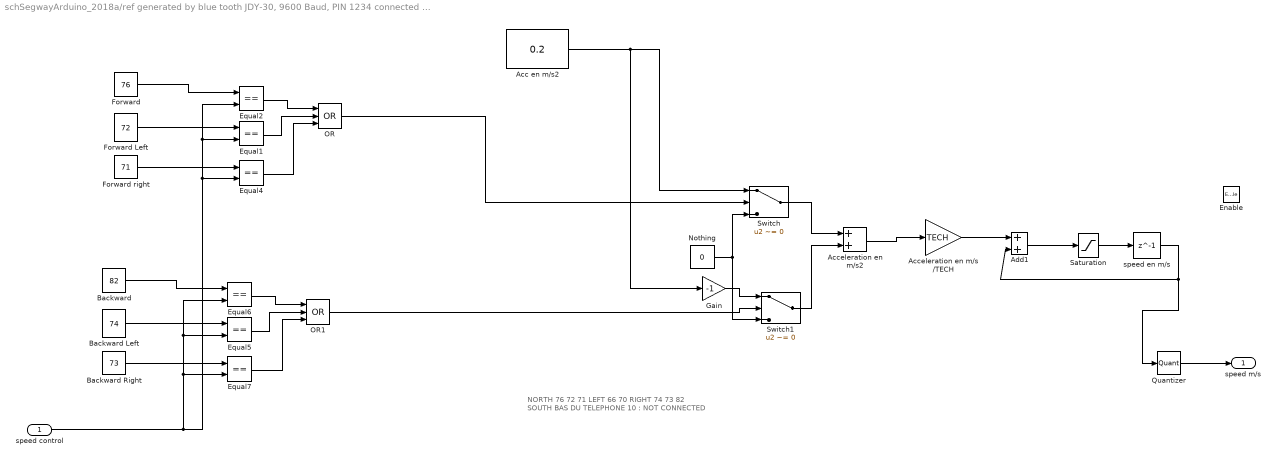
== system schSegwayArduino_2018a/ref generated by blue tooth JDY-30, 9600 Baud, PIN 1234 connected on rx3 pin 15/accelerateur ==
  note: NORTH
      | 				76
      | 			72		71
      | LEFT	66				70	RIGHT
      | 			74		73
      | 				82
      | 			  SOUTH
      |             BAS DU TELEPHONE
      | 10 : NOT CONNECTED
  speed control : Inport
  Enable : EnablePort
  Acc en m/s2 : Constant  Value=0.2
  Acceleration en m/s /TECH : Gain  Gain=TECH
  Acceleration en m/s2 : Sum
  Add1 : Sum
  Backward : Constant  Value=82  OutDataTypeStr=uint8
  Backward Left : Constant  Value=74  OutDataTypeStr=uint8
  Backward Right : Constant  Value=73  OutDataTypeStr=uint8
  Equal{1..2,4..7} (6 alike) : RelationalOperator  Operator===  OutDataTypeStr=boolean  RndMeth=Simplest
  Forward : Constant  Value=76  OutDataTypeStr=uint8
  Forward Left : Constant  Value=72  OutDataTypeStr=uint8
  Forward right : Constant  Value=71  OutDataTypeStr=uint8
  Gain : Gain  Gain=-1
  Nothing : Constant  Value=0  OutDataTypeStr=uint8
  OR : Logic  Operator=OR  Inputs=3  IconShape=distinctive  AllPortsSameDT=off  OutDataTypeStr=boolean
  OR1 : Logic  Operator=OR  Inputs=3  IconShape=distinctive  AllPortsSameDT=off  OutDataTypeStr=boolean
  Quantizer : Quantizer  QuantizationInterval=0.05
  Saturation : Saturate
  Switch : Switch  Criteria=u2 ~= 0
  Switch1 : Switch  Criteria=u2 ~= 0
  speed en m/s : Delay  DelayLength=1  SampleTime=TECH
  speed m/s : Outport  InitialOutput=0
  wires:
  OR1/1 -> Switch1/2
  Switch1/1 -> Acceleration en m/s2/2
  Nothing/1 -> Switch1/3, Switch/3
  speed en m/s/1 -> Quantizer/1, Add1/2
  Switch/1 -> Acceleration en m/s2/1
  Gain/1 -> Switch1/1
  Acceleration en m/s /TECH/1 -> Add1/1
  Acceleration en m/s2/1 -> Acceleration en m/s /TECH/1
  Saturation/1 -> speed en m/s/1
  Acc en m/s2/1 -> Gain/1, Switch/1
  Forward/1 -> Equal2/1
  Add1/1 -> Saturation/1
  Quantizer/1 -> speed m/s/1
  Forward Left/1 -> Equal1/1
  Forward right/1 -> Equal4/1
  Equal2/1 -> OR/1
  Equal1/1 -> OR/2
  Equal4/1 -> OR/3
  OR/1 -> Switch/2
  Equal6/1 -> OR1/1
  Equal7/1 -> OR1/3
  Backward/1 -> Equal6/1
  Equal5/1 -> OR1/2
  speed control/1 -> Equal1/2, Equal2/2, Equal4/2, Equal5/2, Equal6/2, Equal7/2
  Backward Left/1 -> Equal5/1
  Backward Right/1 -> Equal7/1

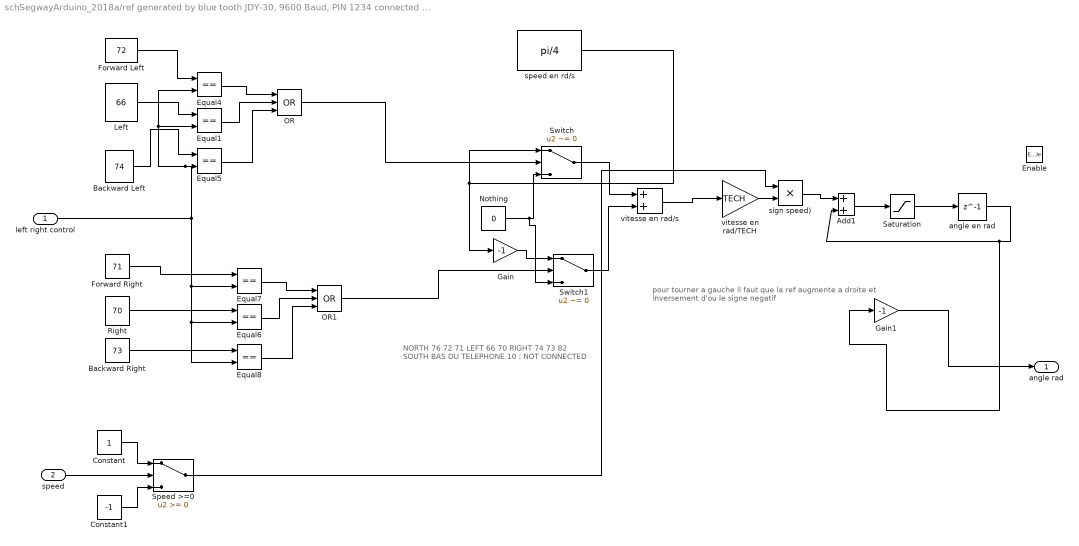
== system schSegwayArduino_2018a/ref generated by blue tooth JDY-30, 9600 Baud, PIN 1234 connected on rx3 pin 15/volant ==
  note: pour tourner a gauche il faut que la ref augmente a droite
      | et inversement
      | d'ou le signe negatif
  note: NORTH
      | 				76
      | 			72		71
      | LEFT	66				70	RIGHT
      | 			74		73
      | 				82
      | 			  SOUTH
      |             BAS DU TELEPHONE
      | 10 : NOT CONNECTED
  left right control : Inport
  speed : Inport  Port=2
  Enable : EnablePort
  Add1 : Sum
  Backward Left : Constant  Value=74  OutDataTypeStr=uint8
  Backward Right : Constant  Value=73  OutDataTypeStr=uint8
  Constant : Constant
  Constant1 : Constant  Value=-1
  Equal{1,4..8} (6 alike) : RelationalOperator  Operator===  OutDataTypeStr=boolean  RndMeth=Simplest
  "Forward Left " : Constant  Value=72  OutDataTypeStr=uint8
  Forward Right : Constant  Value=71  OutDataTypeStr=uint8
  Gain : Gain  Gain=-1
  Gain1 : Gain  Gain=-1
  Left : Constant  Value=66  OutDataTypeStr=uint8
  Nothing : Constant  Value=0  OutDataTypeStr=uint8
  OR : Logic  Operator=OR  Inputs=3  IconShape=distinctive  AllPortsSameDT=off  OutDataTypeStr=boolean
  OR1 : Logic  Operator=OR  Inputs=3  IconShape=distinctive  AllPortsSameDT=off  OutDataTypeStr=boolean
  "Right " : Constant  Value=70  OutDataTypeStr=uint8
  Saturation : Saturate  UpperLimit=1e9*2*pi  LowerLimit=-1e9*2*pi
  Speed >=0 : Switch
  Switch : Switch  Criteria=u2 ~= 0
  Switch1 : Switch  Criteria=u2 ~= 0
  angle en rad : Delay  DelayLength=1  SampleTime=TECH
  sign speed) : Product  Inputs=**
  speed en rd/s : Constant  Value=pi/4
  vitesse en rad/TECH : Gain  Gain=TECH
  vitesse en rad/s : Sum
  angle rad : Outport  InitialOutput=0
  wires:
  Add1/1 -> Saturation/1
  Switch1/1 -> vitesse en rad/s/2
  Nothing/1 -> Switch1/3, Switch/3
  Switch/1 -> vitesse en rad/s/1
  Gain/1 -> Switch1/1
  vitesse en rad/s/1 -> vitesse en rad/TECH/1
  Saturation/1 -> angle en rad/1
  speed en rd/s/1 -> Switch/1, Gain/1
  vitesse en rad/TECH/1 -> sign speed)/2
  sign speed)/1 -> Add1/1
  speed/1 -> Speed >=0/2
  Speed >=0/1 -> sign speed)/1
  Constant/1 -> Speed >=0/1
  Constant1/1 -> Speed >=0/3
  Backward Left/1 -> Equal5/1
  Left/1 -> Equal1/1
  Equal8/1 -> OR1/3
  "Forward Left "/1 -> Equal4/1
  Equal6/1 -> OR1/2
  Forward Right/1 -> Equal7/1
  Equal4/1 -> OR/1
  Equal5/1 -> OR/3
  "Right "/1 -> Equal6/1
  Equal7/1 -> OR1/1
  left right control/1 -> Equal8/2, Equal6/2, Equal7/2, Equal1/2, Equal4/2, Equal5/2
  Equal1/1 -> OR/2
  Backward Right/1 -> Equal8/1
  OR/1 -> Switch/2
  OR1/1 -> Switch1/2
  Gain1/1 -> angle rad/1
  angle en rad/1 -> Gain1/1, Add1/2
